simulink model "QuadModel"  (R2014a)
settings: Solver=ode45  StartTime=0.0  StopTime=10.0  RelTol=1e-3
libraries: simulink x8
settings Model: Creator=KOUSTA  LastModifiedBy=KOUSTA
settings DebuggingCC: UnderspecifiedInitializationDetection=Classic

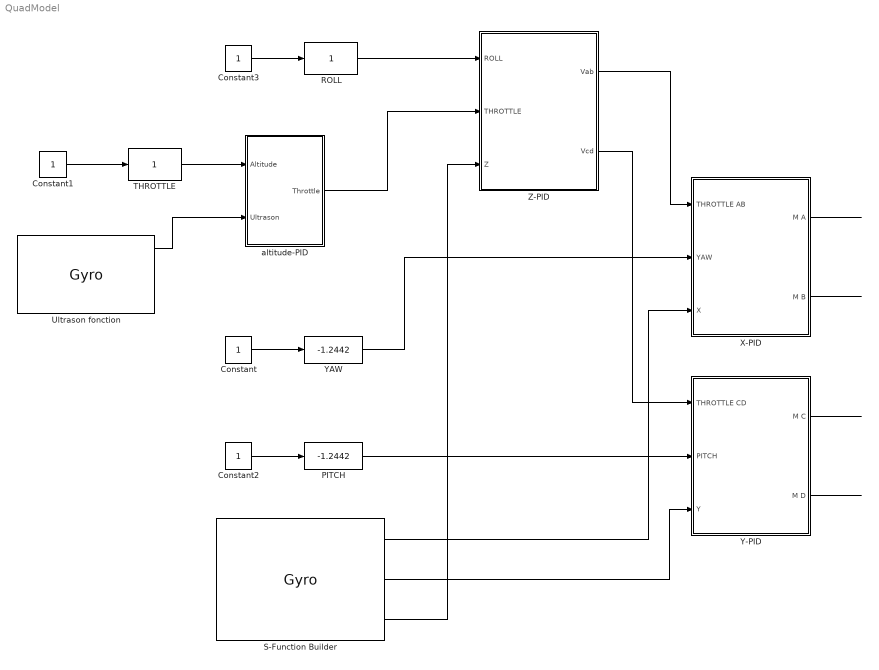
== system QuadModel ==
  Constant{,1..3} (4 alike) : Constant
  PITCH : simulink/Math Operations/Slider Gain  low=-90  gain=-1.2442  high=90
  ROLL : simulink/Math Operations/Slider Gain  low=0  gain=1  high=120
  S-Function Builder : S-Function  InitFcn=try, set_param(gcb,'FunctionName','Gyro'), end  FunctionName=Gyro  SFunctionModules=Gyro_wrapper  EnableBusSupport=off  mask(S-Function Builder){}
      mask help: Simulink:masks:SFunctionBuilder_MD
      mask init:
      | val = [[.9  0.75 0.75 1 1 .9 .9 1]',[1 1 0.75 0.75 .9 .9 1 .9]'];try , sys = get_param(gcb,'SfunBuilderFcnName');if isempty(sys), sys = get_param(gcb,'FunctionName'); end,catch, sys = get_param(gcb,'FunctionName'); end
      settings: CopyFcn=set_param(gcbh,'LinkStatus','none')  PreSaveFcn=try, set_param(gcb,'FunctionName','Gyro'), end  OpenFcn=sfunctionwizard(gcbh)
      mask Display: plot(val(:,1),val(:,2)),disp(sys), port_label('output',1,'X'), port_label('output',2,'Y'), port_label('output',3,'Z')
  THROTTLE : simulink/Math Operations/Slider Gain  low=0  gain=1  high=120
  Ultrason fonction : S-Function  InitFcn=try, set_param(gcb,'FunctionName','Ultrason'), end  FunctionName=Gyro  SFunctionModules=Gyro_wrapper  EnableBusSupport=off  mask(S-Function Builder){}
      mask help: Simulink:masks:SFunctionBuilder_MD
      mask init: same as QuadModel/S-Function Builder
      settings: CopyFcn=set_param(gcbh,'LinkStatus','none')  PreSaveFcn=try, set_param(gcb,'FunctionName','Gyro'), end  OpenFcn=sfunctionwizard(gcbh)
      mask Display: plot(val(:,1),val(:,2)),disp(sys), port_label('output',1,'Distance')
  X-PID : Subsystem
  Y-PID : Subsystem
  YAW : simulink/Math Operations/Slider Gain  low=-90  gain=-1.2442  high=90
  Z-PID : Subsystem
  altitude-PID : Subsystem
  wires:
  Constant/1 -> YAW/1
  Constant1/1 -> THROTTLE/1
  YAW/1 -> X-PID/2(YAW)
  S-Function Builder/1 -> X-PID/3(X)
  X-PID/1(M A) -> ?
  X-PID/2(M B) -> ?
  S-Function Builder/2 -> Y-PID/3(Y)
  Y-PID/1(M C) -> ?
  Y-PID/2(M D) -> ?
  Constant2/1 -> PITCH/1
  PITCH/1 -> Y-PID/2(PITCH)
  Constant3/1 -> ROLL/1
  Z-PID/1(Vab) -> X-PID/1(THROTTLE AB)
  Z-PID/2(Vcd) -> Y-PID/1(THROTTLE CD)
  ROLL/1 -> Z-PID/1(ROLL)
  S-Function Builder/3 -> Z-PID/3(Z)
  altitude-PID/1(Throttle) -> Z-PID/2(THROTTLE)
  THROTTLE/1 -> altitude-PID/1(Altitude)
  Ultrason fonction/1 -> altitude-PID/2(Ultrason)

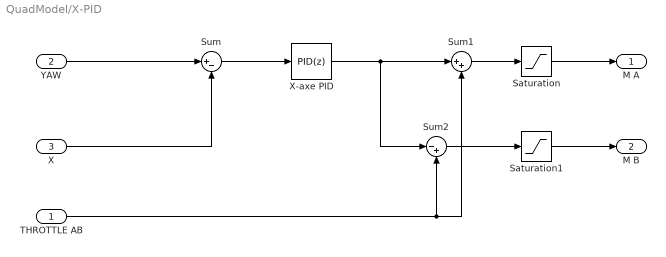
== system QuadModel/X-PID ==
  THROTTLE AB : Inport
  YAW : Inport  Port=2
  X : Inport  Port=3
  Saturation : Saturate
  Saturation1 : Saturate
  Sum : Sum  Inputs=|+-
  Sum1 : Sum  Inputs=|++
  Sum2 : Sum  Inputs=|-+
  X-axe PID : simulink/Continuous/PID Controller  Controller=PID  TimeDomain=Discrete-time  SampleTime=1  IntegratorMethod=Forward Euler  FilterMethod=Forward Euler  Form=Parallel  P=1  I=1  D=0  N=100  InitialConditionSource=internal  InitialConditionForIntegrator=0  InitialConditionForFilter=0  ExternalReset=none  LimitOutput=off  UpperSaturationLimit=inf  LowerSaturationLimit=-inf  LinearizeAsGain=off  AntiWindupMode=none  Kb=1  TrackingMode=off  Kt=1  PParamMin=[]  PParamMax=[]  IParamMin=[]  IParamMax=[]  DParamMin=[]  DParamMax=[]  NParamMin=[]  NParamMax=[]  KbParamMin=[]  KbParamMax=[]  KtParamMin=[]  KtParamMax=[]  POutMin=[]  POutMax=[]  IOutMin=[]  IOutMax=[]  DOutMin=[]  DOutMax=[]  NOutMin=[]  NOutMax=[]  KbOutMin=[]  KbOutMax=[]  KtOutMin=[]  KtOutMax=[]  IntegratorOutMin=[]  IntegratorOutMax=[]  FilterOutMin=[]  FilterOutMax=[]  SumOutMin=[]  SumOutMax=[]  SumI1OutMin=[]  SumI1OutMax=[]  SumI2OutMin=[]  SumI2OutMax=[]  SumI3OutMin=[]  SumI3OutMax=[]  SumDOutMin=[]  SumDOutMax=[]  SaturationOutMin=[]  SaturationOutMax=[]  IntegratorContinuousStateAttributes=''  IntegratorStateMustResolveToSignalObject=off  IntegratorRTWStateStorageClass=Auto  FilterContinuousStateAttributes=''  FilterStateMustResolveToSignalObject=off  FilterRTWStateStorageClass=Auto
  M A : Outport
  M B : Outport  Port=2
  wires:
  Sum/1 -> X-axe PID/1
  Sum1/1 -> Saturation/1
  X-axe PID/1 -> Sum2/1, Sum1/1
  Sum2/1 -> Saturation1/1
  X/1 -> Sum/2
  YAW/1 -> Sum/1
  THROTTLE AB/1 -> Sum1/2, Sum2/2
  Saturation/1 -> M A/1
  Saturation1/1 -> M B/1

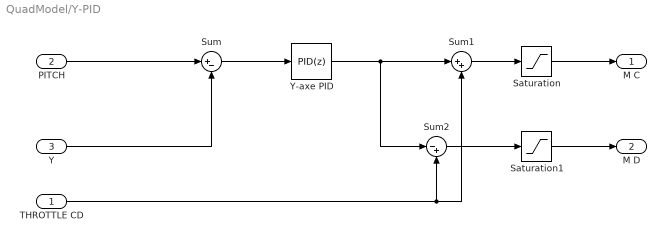
== system QuadModel/Y-PID ==
  THROTTLE CD : Inport
  PITCH : Inport  Port=2
  Y : Inport  Port=3
  Saturation : Saturate
  Saturation1 : Saturate
  Sum : Sum  Inputs=|+-
  Sum1 : Sum  Inputs=|++
  Sum2 : Sum  Inputs=|-+
  Y-axe PID : simulink/Continuous/PID Controller  Controller=PID  TimeDomain=Discrete-time  SampleTime=1  IntegratorMethod=Forward Euler  FilterMethod=Forward Euler  Form=Parallel  P=1  I=1  D=0  N=100  InitialConditionSource=internal  InitialConditionForIntegrator=0  InitialConditionForFilter=0  ExternalReset=none  LimitOutput=off  UpperSaturationLimit=inf  LowerSaturationLimit=-inf  LinearizeAsGain=off  AntiWindupMode=none  Kb=1  TrackingMode=off  Kt=1  PParamMin=[]  PParamMax=[]  IParamMin=[]  IParamMax=[]  DParamMin=[]  DParamMax=[]  NParamMin=[]  NParamMax=[]  KbParamMin=[]  KbParamMax=[]  KtParamMin=[]  KtParamMax=[]  POutMin=[]  POutMax=[]  IOutMin=[]  IOutMax=[]  DOutMin=[]  DOutMax=[]  NOutMin=[]  NOutMax=[]  KbOutMin=[]  KbOutMax=[]  KtOutMin=[]  KtOutMax=[]  IntegratorOutMin=[]  IntegratorOutMax=[]  FilterOutMin=[]  FilterOutMax=[]  SumOutMin=[]  SumOutMax=[]  SumI1OutMin=[]  SumI1OutMax=[]  SumI2OutMin=[]  SumI2OutMax=[]  SumI3OutMin=[]  SumI3OutMax=[]  SumDOutMin=[]  SumDOutMax=[]  SaturationOutMin=[]  SaturationOutMax=[]  IntegratorContinuousStateAttributes=''  IntegratorStateMustResolveToSignalObject=off  IntegratorRTWStateStorageClass=Auto  FilterContinuousStateAttributes=''  FilterStateMustResolveToSignalObject=off  FilterRTWStateStorageClass=Auto
  M C : Outport
  M D : Outport  Port=2
  wires:
  Y/1 -> Sum/2
  Sum2/1 -> Saturation1/1
  Y-axe PID/1 -> Sum1/1, Sum2/1
  Sum1/1 -> Saturation/1
  Sum/1 -> Y-axe PID/1
  THROTTLE CD/1 -> Sum1/2, Sum2/2
  PITCH/1 -> Sum/1
  Saturation/1 -> M C/1
  Saturation1/1 -> M D/1

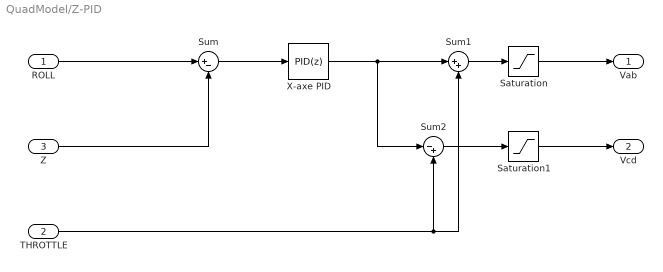
== system QuadModel/Z-PID ==
  ROLL : Inport
  THROTTLE : Inport  Port=2
  Z : Inport  Port=3
  Saturation : Saturate
  Saturation1 : Saturate
  Sum : Sum  Inputs=|+-
  Sum1 : Sum  Inputs=|++
  Sum2 : Sum  Inputs=|-+
  X-axe PID : simulink/Continuous/PID Controller  Controller=PID  TimeDomain=Discrete-time  SampleTime=1  IntegratorMethod=Forward Euler  FilterMethod=Forward Euler  Form=Parallel  P=1  I=1  D=0  N=100  InitialConditionSource=internal  InitialConditionForIntegrator=0  InitialConditionForFilter=0  ExternalReset=none  LimitOutput=off  UpperSaturationLimit=inf  LowerSaturationLimit=-inf  LinearizeAsGain=off  AntiWindupMode=none  Kb=1  TrackingMode=off  Kt=1  PParamMin=[]  PParamMax=[]  IParamMin=[]  IParamMax=[]  DParamMin=[]  DParamMax=[]  NParamMin=[]  NParamMax=[]  KbParamMin=[]  KbParamMax=[]  KtParamMin=[]  KtParamMax=[]  POutMin=[]  POutMax=[]  IOutMin=[]  IOutMax=[]  DOutMin=[]  DOutMax=[]  NOutMin=[]  NOutMax=[]  KbOutMin=[]  KbOutMax=[]  KtOutMin=[]  KtOutMax=[]  IntegratorOutMin=[]  IntegratorOutMax=[]  FilterOutMin=[]  FilterOutMax=[]  SumOutMin=[]  SumOutMax=[]  SumI1OutMin=[]  SumI1OutMax=[]  SumI2OutMin=[]  SumI2OutMax=[]  SumI3OutMin=[]  SumI3OutMax=[]  SumDOutMin=[]  SumDOutMax=[]  SaturationOutMin=[]  SaturationOutMax=[]  IntegratorContinuousStateAttributes=''  IntegratorStateMustResolveToSignalObject=off  IntegratorRTWStateStorageClass=Auto  FilterContinuousStateAttributes=''  FilterStateMustResolveToSignalObject=off  FilterRTWStateStorageClass=Auto
  Vab : Outport
  Vcd : Outport  Port=2
  wires:
  Sum/1 -> X-axe PID/1
  THROTTLE/1 -> Sum1/2, Sum2/2
  Sum1/1 -> Saturation/1
  X-axe PID/1 -> Sum2/1, Sum1/1
  Sum2/1 -> Saturation1/1
  Z/1 -> Sum/2
  ROLL/1 -> Sum/1
  Saturation/1 -> Vab/1
  Saturation1/1 -> Vcd/1

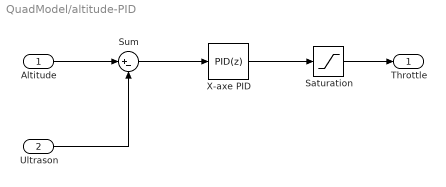
== system QuadModel/altitude-PID ==
  Altitude : Inport
  Ultrason : Inport  Port=2
  Saturation : Saturate
  Sum : Sum  Inputs=|+-
  X-axe PID : simulink/Continuous/PID Controller  Controller=PID  TimeDomain=Discrete-time  SampleTime=1  IntegratorMethod=Forward Euler  FilterMethod=Forward Euler  Form=Parallel  P=1  I=1  D=0  N=100  InitialConditionSource=internal  InitialConditionForIntegrator=0  InitialConditionForFilter=0  ExternalReset=none  LimitOutput=off  UpperSaturationLimit=inf  LowerSaturationLimit=-inf  LinearizeAsGain=off  AntiWindupMode=none  Kb=1  TrackingMode=off  Kt=1  PParamMin=[]  PParamMax=[]  IParamMin=[]  IParamMax=[]  DParamMin=[]  DParamMax=[]  NParamMin=[]  NParamMax=[]  KbParamMin=[]  KbParamMax=[]  KtParamMin=[]  KtParamMax=[]  POutMin=[]  POutMax=[]  IOutMin=[]  IOutMax=[]  DOutMin=[]  DOutMax=[]  NOutMin=[]  NOutMax=[]  KbOutMin=[]  KbOutMax=[]  KtOutMin=[]  KtOutMax=[]  IntegratorOutMin=[]  IntegratorOutMax=[]  FilterOutMin=[]  FilterOutMax=[]  SumOutMin=[]  SumOutMax=[]  SumI1OutMin=[]  SumI1OutMax=[]  SumI2OutMin=[]  SumI2OutMax=[]  SumI3OutMin=[]  SumI3OutMax=[]  SumDOutMin=[]  SumDOutMax=[]  SaturationOutMin=[]  SaturationOutMax=[]  IntegratorContinuousStateAttributes=''  IntegratorStateMustResolveToSignalObject=off  IntegratorRTWStateStorageClass=Auto  FilterContinuousStateAttributes=''  FilterStateMustResolveToSignalObject=off  FilterRTWStateStorageClass=Auto
  Throttle : Outport
  wires:
  Saturation/1 -> Throttle/1
  Altitude/1 -> Sum/1
  Ultrason/1 -> Sum/2
  X-axe PID/1 -> Saturation/1
  Sum/1 -> X-axe PID/1
